simulink model "fin_simu"  (R2022a)
settings: Solver=FixedStepDiscrete  StartTime=0.0  StopTime=time  FixedStep=ts  RelTol=1e-6
values from neighbouring files (symbols this model uses):
  A = [0.7, 0.2; 0, 0.5]    [code_simu.m]    (also in code_simu_continuous.m)
  A0 = [0, 1; -1, -1.4]    [code_simu_continuous.m]
  B = [1; 0.5]    [code_simu.m]    (also in code_simu_continuous.m)
  B0 = [0; 1]    [code_simu_continuous.m]
  C = [0.2, 0.8]    [code_simu.m]    (also in code_simu_continuous.m)
  C0 = [1, 0]    [code_simu_continuous.m]
  D = [0]    [code_simu.m]    (also in code_simu_continuous.m)
  D0 = [0]    [code_simu_continuous.m]
  gamma = 2    [code_simu.m]    (also in code_simu_continuous.m)
  omega = 3.14159265*5    (= 15.70796325)    [code_simu.m]    (also in code_simu_continuous.m)
  ran_max = 20    [code_simu.m]    (also in code_simu_continuous.m)
  ran_min = 5    [code_simu.m]    (also in code_simu_continuous.m)
  rho = 0.101    [code_simu.m]    (also in code_simu_continuous.m)
  sam_time = 40    [code_simu.m]    (also in code_simu_continuous.m)
  seed = 17    [code_simu.m]    (also in code_simu_continuous.m)
  sig = 0.001    [code_simu.m]    (also in code_simu_continuous.m)
  sigma = 10    [code_simu.m]    (also in code_simu_continuous.m)
  ts = 0.005    [code_simu.m]    (also in code_simu_continuous.m)
  wav = 0.7    [code_simu.m]    (also in code_simu_continuous.m)
undefined symbols (not defined in the file or in its folder): A_aspr, AA, b0, b0pfc, b1, b1pfc, b2, b2pfc, b3, b3pfc, B_aspr, BB, C_aspr, CC, D_aspr, DD, w0, w0pfc, w1, w1pfc, w2, w2pfc, w3, w3pfc
libraries: matrix_library x1
settings Model: Creator=lenovo  LastModifiedBy=IDS_PC
settings ModelReferenceCC: EnableRefExpFcnMdlSchedulingChecks=off
settings RTWCC: Description=Generic Real-Time Target  GPUComputeCapability=5.0

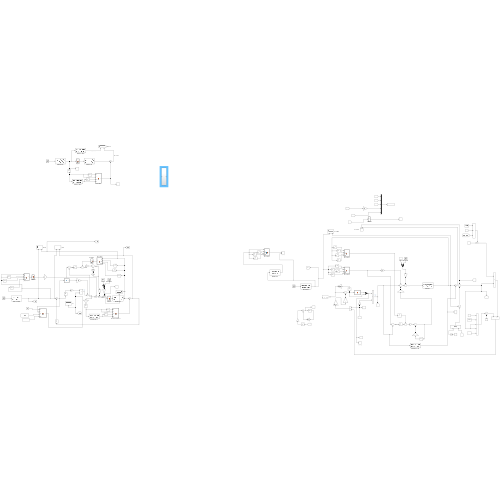
[thumbnail: Simulink's stored preview of the top-level diagram]
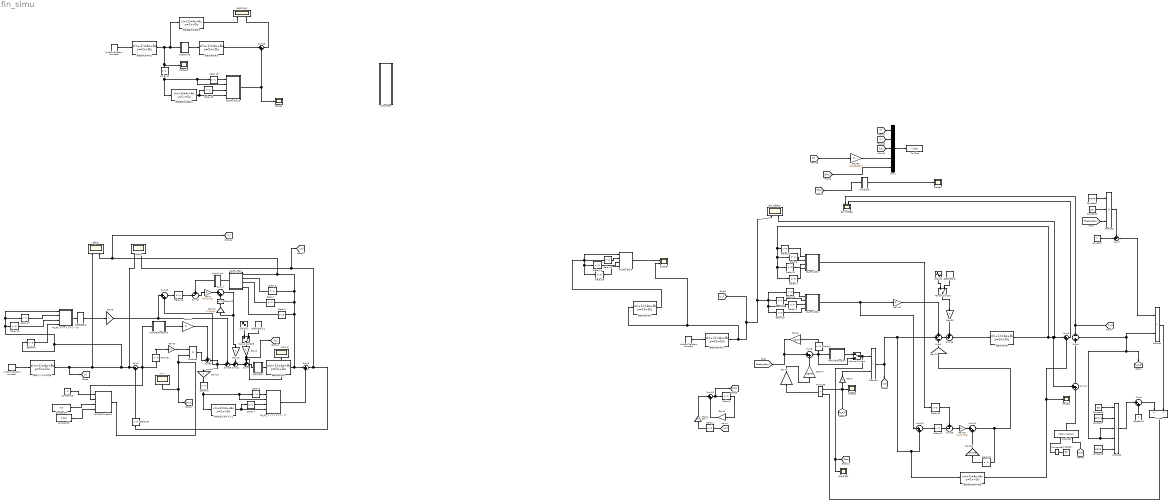
== system fin_simu ==
  " 正弦外乱" : Sin  Amplitude=wav  Frequency=omega  SampleTime=ts
  " 正弦外乱1" : Sin  Amplitude=wav  Frequency=omega  SampleTime=ts
  Constant : Constant  SampleTime=ts
  Constant1 : Constant  Value=sigma  SampleTime=ts
  Constant10 : Constant  Value=0  SampleTime=ts
  Constant14 : Constant  Value=0.5  SampleTime=ts
  Constant15 : Constant  Value=0.001  SampleTime=ts
  Constant2 : Constant  Value=DD  SampleTime=ts
  Constant3 : Constant  Value=sigma  SampleTime=ts
  Constant4 : Constant  SampleTime=ts
  Constant6 : Constant  Value=DD  SampleTime=ts
  Constant7 : Constant  Value=gamma  SampleTime=ts
  Constant8 : Constant  Value=CC  SampleTime=ts
  Delay{1..6,8,12,14,20..23,42..45,47} (18 alike) : Delay  DelayLength=1  InitialCondition=0  SampleTime=ts
  Delay{7,10..11,13,48} (5 alike) : Delay  InitialCondition=0  SampleTime=ts
  Delay{15..16,40,50..51} (5 alike) : Delay  DelayLength=0  InitialCondition=0  SampleTime=ts
  Delay{9,17..19,49} (5 alike) : Delay  DelayLength=3  InitialCondition=0  SampleTime=ts
  Divide : Product  Inputs=/*
  Gain1 : Gain  Gain=BB  Multiplication=Matrix(K*u)
  Gain{5,9..10,12} (4 alike) : Gain
  Gain11 : Gain  Gain=1/(1+sig)
  Gain14 : Gain  Gain=sigma
  Gain{15,21,35,40} (4 alike) : Gain  Gain=0
  Gain2 : Gain  Gain=-1
  Gain3 : Gain  Gain=AA  Multiplication=Matrix(K*u)
  Gain36 : Gain  Gain=1/(1+sig)
  Gain37 : Gain  Gain=rho/(1+sig)
  Gain39 : Gain  Gain=16.66666667
  Gain4 : Gain  Gain=gamma
  Gain6 : Gain  Gain=sigma
  Gain7 : Gain  Gain=rho/(1+sig)
  Gain8 : Gain  Gain=-1
  MATLAB Function : MATLAB Function  TreatAsAtomicUnit=on
  MATLAB Function3 : MATLAB Function  TreatAsAtomicUnit=on
  MATLAB Function4 : MATLAB Function  TreatAsAtomicUnit=on
  Manual Switch1 : ManualSwitch  CurrentSetting=0
  Manual Switch4 : ManualSwitch
  Manual Switch5 : ManualSwitch  CurrentSetting=0
  Mux2 : Mux  Inputs=5
  NNPFC验证 : Scope  NumInputPorts=2
  NN_FF_フィードフォワード7 : MATLAB Function  TreatAsAtomicUnit=on
  NN_FF_フィードフォワード9 : MATLAB Function  TreatAsAtomicUnit=on
  NN_FF_前馈1 : MATLAB Function  TreatAsAtomicUnit=on
  NN_FF_前馈10 : MATLAB Function  TreatAsAtomicUnit=on
  NN_FF_前馈3 : MATLAB Function  TreatAsAtomicUnit=on
  NN_FF_前馈5 : MATLAB Function  TreatAsAtomicUnit=on
  NN_FF_前馈6 : MATLAB Function  TreatAsAtomicUnit=on
  PFC输出 : Scope
  Product{,2,4..5} (4 alike) : Product
  Product1 : Product  Inputs=3
  Product3 : Product  Inputs=5
  Product6 : Product  Multiplication=Matrix(*)
  Scope{1..2,5,10} (4 alike) : Scope
  Subsystem : Subsystem
  Sum1 : Sum  Inputs=|-+
  Sum{4,10,16,28,33} (5 alike) : Sum  Inputs=++|
  Sum11 : Sum  Inputs=-+|
  Sum{2,5,8..9,12..13,15,17,22,24} (10 alike) : Sum  Inputs=|++
  Sum14 : Sum  Inputs=+-|
  Sum23 : Sum  Inputs=+-|
  Sum3 : Sum  Inputs=++-
  Sum6 : Sum  Inputs=-|+
  Sum7 : Sum  Inputs=-+|
  To File2 : ToFile  Filename=linear  MatrixName=linear  SampleTime=ts
  Transpose : matrix_library/Transpose
      settings: SourceProductBaseCode=SL
  Uniform Random Number1 : UniformRandomNumber  Minimum=ran_min  Maximum=ran_max  Seed=seed  SampleTime=sam_time
  Uniform Random Number2 : UniformRandomNumber  Minimum=5  Maximum=20  Seed=seed  SampleTime=sam_time
  Uniform Random Number3 : UniformRandomNumber  Minimum=0  Seed=seed  SampleTime=sam_time
  wailuan : Scope
  ゲイン : Scope
  代号返回器 : MATLAB Function  TreatAsAtomicUnit=on
  伪输出 : Scope  NumInputPorts=2
  拟合效果 : Scope  NumInputPorts=2
  理想拡張正実モデル1 : DiscreteStateSpace  A=A_aspr  B=B_aspr  C=C_aspr  D=D_aspr  SampleTime=ts
  理想概强正实模型2 : DiscreteStateSpace  A=A_aspr  B=B_aspr  C=C_aspr  D=D_aspr  SampleTime=ts
  理想概强正实模型3 : DiscreteStateSpace  A=A_aspr  B=B_aspr  C=C_aspr  D=D_aspr  SampleTime=ts
  真输出1 : Scope  NumInputPorts=2
  离散初始信号机1 : DiscreteStateSpace  A=A0  B=B0  C=C0  D=D0  SampleTime=ts
  离散控制对象 : DiscreteStateSpace  A=A  B=B  C=C  D=D  SampleTime=ts
  离散控制对象2 : DiscreteStateSpace  A=A  B=B  C=C  D=D  SampleTime=ts
  离散控制对象3 : DiscreteStateSpace  A=A  B=B  C=C  D=D  SampleTime=ts
  离散理想前馈补偿器 : DiscreteStateSpace  A=AA  B=BB  C=CC  D=DD  SampleTime=ts
  离散随机信号机1 : DiscreteStateSpace  A=A0  B=B0  C=C0  D=D0  SampleTime=ts
  自适应增益 : Scope
  输入与伪输出 : Scope  NumInputPorts=2
  输入与真输出 : Scope  NumInputPorts=2
  随机阶梯外乱 : UniformRandomNumber  Minimum=-wav  Maximum=wav  Seed=seed+5  SampleTime=16
  随机阶梯外乱1 : UniformRandomNumber  Minimum=-wav  Maximum=wav  Seed=seed+5  SampleTime=16
  離散ランダム信号機 : DiscreteStateSpace  A=A0  B=B0  C=C0  D=D0  SampleTime=ts
  離散制御対象1 : DiscreteStateSpace  A=A  B=B  C=C  D=D  SampleTime=ts
  非線形要素6 : MATLAB Function  TreatAsAtomicUnit=on
  非線形要素7 : MATLAB Function  TreatAsAtomicUnit=on
  非线性元件4 : MATLAB Function  TreatAsAtomicUnit=on
  非线性元件5 : MATLAB Function  TreatAsAtomicUnit=on
  wires:
  Uniform Random Number1/1 -> 离散初始信号机1/1
  Sum6/1 -> Product/2, [e_a_2], Product3/4, Product3/3
  Product1/1 -> Sum7/1
  Constant/1 -> Sum7/2
  Sum7/1 -> Product/1
  Constant1/1 -> Product1/1
  Gain2/1 -> Product4/2
  Sum9/1 -> Manual Switch4/2, Delay2/1, MATLAB Function/1(k)
  Gain6/1 -> Sum9/1, [theta_delay]
  [y_r] -> Sum6/1, 输入与伪输出/1
  Product/1 -> Divide/2
  Sum8/1 -> Divide/1
  Product3/1 -> Sum8/1
  Constant4/1 -> Sum8/2
  Constant7/1 -> Product3/2
  Sum10/1 -> Sum6/2
  [u2] -> Delay1/1
  Delay1/1 -> Gain1/1
  Delay3/1 -> Gain3/1
  Gain3/1 -> Sum12/2
  Sum12/1 -> [xf_k], Delay3/1
  [xf_k] -> Product6/2
  Gain1/1 -> Sum12/1
  Transpose/1 -> Product6/1
  Constant8/1 -> Transpose/1
  Sum5/1 -> Delay50/1, [ya], 伪输出/2
  Uniform Random Number2/1 -> 離散ランダム信号機/1
  離散ランダム信号機/1 -> [r], 伪输出/1, Sum1/1, Delay47/1, NN_FF_フィードフォワード9/1(y), Delay48/1, Delay49/1, 真输出1/1
  [e_a_2] -> Scope5/1, Gain2/1, Product5/1
  [theta_delay] -> Product1/3
  Constant2/1 -> Product1/2
  Constant6/1 -> Product3/1
  Product5/1 -> Gain4/1
  Constant3/1 -> Product3/5
  Gain4/1 -> Gain14/1
  Gain14/1 -> Sum9/2
  Divide/1 -> Product5/2
  Sum16/1 -> 离散控制对象/1  "外乱输入"
  Gain15/1 -> Sum3/1
  Delay2/1 -> Gain6/1
  Product6/1 -> Sum10/2
  Delay8/1 -> NN_FF_前馈3/2(yd)
  Delay10/1 -> NN_FF_前馈3/3(ydd)
  离散控制对象2/1 -> NN_FF_前馈5/1(y), Delay13/1, Delay19/1, Delay14/1
  Delay13/1 -> NN_FF_前馈5/3(ydd)
  Delay14/1 -> NN_FF_前馈5/2(yd)
  NN_FF_前馈5/1(v) -> 拟合效果/1
  Delay15/1 -> NN_FF_前馈3/1(y)
  Delay17/1 -> NN_FF_前馈3/4(yddd)
  Delay16/1 -> NN_FF_前馈6/1(y)
  Delay12/1 -> NN_FF_前馈6/2(yd)
  Delay11/1 -> NN_FF_前馈6/3(ydd)
  Delay18/1 -> NN_FF_前馈6/4(yddd)
  Delay19/1 -> NN_FF_前馈5/4(yddd)
  Manual Switch1/1 -> Gain35/1
  随机阶梯外乱/1 -> Manual Switch1/2
  " 正弦外乱"/1 -> Manual Switch1/1
  离散理想前馈补偿器/1 -> Sum2/2, PFC输出/1
  Sum3/1 -> Sum16/2
  MATLAB Function/1(y) -> Manual Switch4/1
  Product4/1 -> Sum3/2, Sum22/2, 离散理想前馈补偿器/1, [u2]
  离散控制对象/1 -> Delay17/1, Delay10/1, Delay8/1, Delay15/1, Sum2/1, 输入与真输出/2, Sum10/1
  NN_FF_前馈3/1(v) -> Delay40/1
  Gain21/1 -> Sum3/3
  Sum24/1 -> Gain21/1, Delay22/1
  Manual Switch4/1 -> 自适应增益/1, [the], Product4/1
  Sum22/1 -> Delay21/1  "外乱输入"
  Delay21/1 -> Sum23/2
  Sum23/1 -> Gain37/1
  Delay22/1 -> Gain36/1
  离散初始信号机1/1 -> Delay12/1, Delay18/1, Delay11/1, Delay16/1, 输入与真输出/1, [y_r], 拟合效果/2, 离散控制对象2/1
  Delay40/1 -> Sum23/1
  Gain35/1 -> Sum16/1
  NN_FF_前馈6/1(v) -> Sum22/1, Gain15/1
  Gain36/1 -> Sum24/2
  Gain37/1 -> Sum24/1
  非線形要素7/1(y) -> 離散制御対象1/1
  理想拡張正実モデル1/1 -> Delay4/1, NN_FF_フィードフォワード7/4(ya)
  Delay4/1 -> NN_FF_フィードフォワード7/3(ya1)
  Delay5/1 -> NN_FF_フィードフォワード7/1(u1)
  NN_FF_フィードフォワード7/1(v) -> Sum5/2
  Gain8/1 -> Product2/1
  Delay42/1 -> NN_FF_フィードフォワード7/2(u), Delay5/1, 理想拡張正実モデル1/1
  Delay44/1 -> NN_FF_前馈10/2(u), Delay45/1, 理想概强正实模型2/1
  理想概强正实模型2/1 -> NN_FF_前馈10/4(ya), Delay43/1
  Delay43/1 -> NN_FF_前馈10/3(ya1)
  Delay45/1 -> NN_FF_前馈10/1(u1)
  非线性元件5/1(y) -> 离散控制对象3/1
  Uniform Random Number3/1 -> 离散随机信号机1/1
  离散控制对象3/1 -> Sum15/1
  NN_FF_前馈10/1(v) -> Scope2/1, Sum15/2
  理想概强正实模型3/1 -> NNPFC验证/1  "理想扩张输出"
  Sum15/1 -> NNPFC验证/2  "真实扩张输出"
  Mux2/1 -> To File2/1
  [ya] -> Mux2/3
  [r] -> Mux2/1
  [y] -> Mux2/2
  [d] -> Gain39/1
  [the] -> 代号返回器/1(u)
  代号返回器/1(y) -> Scope1/1
  NN_FF_フィードフォワード9/1(v) -> 非線形要素6/1(u)
  Delay47/1 -> NN_FF_フィードフォワード9/2(yd)
  Delay48/1 -> NN_FF_フィードフォワード9/3(ydd)
  Delay49/1 -> NN_FF_フィードフォワード9/4(yddd)
  非線形要素6/1(y) -> Gain9/1
  Gain10/1 -> Delay42/1
  離散制御対象1/1 -> Sum5/1, Delay7/1, [y], 真输出1/2, NN_FF_前馈1/1(y), Delay6/1, Delay9/1
  离散随机信号机1/1 -> Delay44/1, Scope10/1, 理想概强正实模型3/1, 非线性元件5/1(u)
  Delay50/1 -> Sum1/2
  Delay51/1 -> Gain8/1
  Sum2/1 -> 输入与伪输出/2
  Gain39/1 -> Mux2/4
  Constant10/1 -> MATLAB Function4/1(ht)
  Sum1/1 -> MATLAB Function4/2(e), MATLAB Function3/1(e), Delay51/1
  Constant14/1 -> MATLAB Function4/3(sig)
  Constant15/1 -> MATLAB Function4/4(gam)
  MATLAB Function4/1(y) -> ゲイン/1, [thno], Product2/2
  Sum33/1 -> Sum13/2, Sum28/2, Gain10/1
  Product2/1 -> Sum33/2
  MATLAB Function3/1(y) -> Gain40/1
  Gain40/1 -> Sum33/1
  NN_FF_前馈1/1(v) -> 非线性元件4/1(u)
  Manual Switch5/1 -> Gain5/1
  随机阶梯外乱1/1 -> Manual Switch5/2
  " 正弦外乱1"/1 -> Manual Switch5/1
  Sum4/1 -> 非線形要素7/1(u)
  Gain5/1 -> [d], wailuan/1, Sum4/1
  Gain9/1 -> Sum13/1, Sum28/1
  Delay6/1 -> NN_FF_前馈1/2(yd)
  Delay7/1 -> NN_FF_前馈1/3(ydd)
  Delay9/1 -> NN_FF_前馈1/4(yddd)
  Sum11/1 -> Sum4/2  "外乱输入"
  Sum28/1 -> Sum11/2
  Sum13/1 -> Delay20/1  "外乱输入"
  Delay20/1 -> Sum14/2
  非线性元件4/1(y) -> Sum14/1
  Sum14/1 -> Gain7/1  "外乱输入"
  Gain7/1 -> Sum17/1
  Sum17/1 -> Gain12/1, Gain11/1  "外乱输入"
  Gain11/1 -> Delay23/1
  Delay23/1 -> Sum17/2
  Gain12/1 -> Sum11/1
  [thno] -> Mux2/5

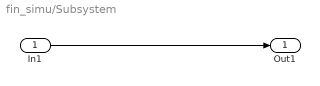
== system fin_simu/Subsystem ==
  In1 : Inport
  Out1 : Outport
  wires:
  In1/1 -> Out1/1

== matlab function fin_simu/NN_FF_フィードフォワード7 ==
  data: u1 input; u input; ya1 input; ya input; v output; w0pfc parameter; w1pfc parameter; w2pfc parameter; w3pfc parameter; b0pfc parameter; b1pfc parameter; b2pfc parameter; b3pfc parameter
function v = fcn(u1, u, ya1, ya, w0pfc, w1pfc, w2pfc, w3pfc, b0pfc, b1pfc, b2pfc, b3pfc)

    x = [ya,ya1,u,u1];
    x = x.';

    s1= (transpose(w0pfc)) * x + b0pfc;
    x1= max(0,s1);     %relu 
    s2= (transpose(w1pfc)) * x1 + b1pfc;
    x2= max(0,s2);     %relu
    s3= (transpose(w2pfc)) * x2 + b2pfc;
    x3= max(0,s3);     %relu
    s4= (transpose(w3pfc)) * x3 + b3pfc;

v=s4;

== matlab function fin_simu/代号返回器 ==
  data: u input; y output
function y = fcn(u)

y = (1+u)/(1-u);
end

== matlab function fin_simu/非线性元件5 ==
  data: u input; y output
function y = fcn(u)

y = 0.06*u^2+0.12*u;
end

== matlab function fin_simu/NN_FF_前馈10 ==
  data: u1 input; u input; ya1 input; ya input; v output; w0pfc parameter; w1pfc parameter; w2pfc parameter; w3pfc parameter; b0pfc parameter; b1pfc parameter; b2pfc parameter; b3pfc parameter
function v = fcn(u1, u, ya1, ya, w0pfc, w1pfc, w2pfc, w3pfc, b0pfc, b1pfc, b2pfc, b3pfc)

    x = [ya,ya1,u,u1];
    x = x.';

    s1= (transpose(w0pfc)) * x + b0pfc;
    x1= max(0,s1);     %relu 
    s2= (transpose(w1pfc)) * x1 + b1pfc;
    x2= max(0,s2);     %relu
    s3= (transpose(w2pfc)) * x2 + b2pfc;
    x3= max(0,s3);     %relu
    s4= (transpose(w3pfc)) * x3 + b3pfc;

v=s4;

== matlab function fin_simu/NN_FF_フィードフォワード9 ==
  data: y input; yd input; ydd input; yddd input; v output; w0 parameter; w1 parameter; w2 parameter; w3 parameter; b0 parameter; b1 parameter; b2 parameter; b3 parameter
function v = fcn(y, yd, ydd, yddd, w0, w1, w2, w3, b0, b1, b2, b3)

    x = [yddd, ydd, yd, y];
    x = x.';

    s1= (transpose(w0)) * x + b0;
    x1= max(0,s1);     %relu 
    s2= (transpose(w1)) * x1 + b1;
    x2= max(0,s2);     %relu
    s3= (transpose(w2)) * x2 + b2;
    x3= max(0,s3);     %relu
    s4= (transpose(w3)) * x3 + b3;

v=s4;

== matlab function fin_simu/非線形要素6 ==
  data: u input; y output
function y = fcn(u)

y = sqrt(u/0.06+1)-1;
end

== matlab function fin_simu/非線形要素7 ==
  data: u input; y output
function y = fcn(u)

y = 0.06*u^2+0.12*u;
end

== matlab function fin_simu/MATLAB Function3 ==
  data: y output; e input
function y = fcn(e)

persistent e_prev;

if isempty(e_prev)
    e_prev = 0;
end

e_next = e_prev + e ;
e_prev = e_next;

y = e_next * 1;

end

== matlab function fin_simu/MATLAB Function4 ==
  data: ht input; y output; e input; sig input; gam input
function y = fcn(ht, e, sig, gam)

persistent k_prev;

if isempty(k_prev)
    k_prev = ht;
end

k_next = k_prev / (1 + sig) + gam / (1 + sig) * e ;
k_prev = k_next;

y = k_next * 1;

end

== matlab function fin_simu/NN_FF_前馈1 ==
  data: y input; yd input; ydd input; yddd input; v output; w0 parameter; w1 parameter; w2 parameter; w3 parameter; b0 parameter; b1 parameter; b2 parameter; b3 parameter
function v = fcn(y, yd, ydd, yddd, w0, w1, w2, w3, b0, b1, b2, b3)

    x = [yddd, ydd, yd, y];
    x = x.';

    s1= (transpose(w0)) * x + b0;
    x1= max(0,s1);     %relu 
    s2= (transpose(w1)) * x1 + b1;
    x2= max(0,s2);     %relu
    s3= (transpose(w2)) * x2 + b2;
    x3= max(0,s3);     %relu
    s4= (transpose(w3)) * x3 + b3;

v=s4;

== matlab function fin_simu/非线性元件4 ==
  data: u input; y output
function y = fcn(u)

y = sqrt(u/0.06+1)-1;
end

== matlab function fin_simu/MATLAB Function ==
  data: y output; k input
function y = fcn(k)

if k>=0 && k<0.999
    y=k;
else
    y=0.998;
end

== matlab function fin_simu/NN_FF_前馈3 ==
  data: y input; yd input; ydd input; yddd input; v output; w0 parameter; w1 parameter; w2 parameter; w3 parameter; b0 parameter; b1 parameter; b2 parameter; b3 parameter
function v = fcn(y, yd, ydd, yddd, w0, w1, w2, w3, b0, b1, b2, b3)

    x = [yddd, ydd, yd, y];
    x = x.';

    s1= (transpose(w0)) * x + b0;
    x1= max(0,s1);     %relu 
    s2= (transpose(w1)) * x1 + b1;
    x2= max(0,s2);     %relu
    s3= (transpose(w2)) * x2 + b2;
    x3= max(0,s3);     %relu
    s4= (transpose(w3)) * x3 + b3;

v=s4;

== matlab function fin_simu/NN_FF_前馈5 ==
  data: y input; yd input; ydd input; yddd input; v output; w0 parameter; w1 parameter; w2 parameter; w3 parameter; b0 parameter; b1 parameter; b2 parameter; b3 parameter
function v = fcn(y, yd, ydd, yddd, w0, w1, w2, w3, b0, b1, b2, b3)

    x = [yddd, ydd, yd, y];
    x = x.';

    s1= (transpose(w0)) * x + b0;
    x1= max(0,s1);     %relu 
    s2= (transpose(w1)) * x1 + b1;
    x2= max(0,s2);     %relu
    s3= (transpose(w2)) * x2 + b2;
    x3= max(0,s3);     %relu
    s4= (transpose(w3)) * x3 + b3;

v=s4;

== matlab function fin_simu/NN_FF_前馈6 ==
  data: y input; yd input; ydd input; yddd input; v output; w0 parameter; w1 parameter; w2 parameter; w3 parameter; b0 parameter; b1 parameter; b2 parameter; b3 parameter
function v = fcn(y, yd, ydd, yddd, w0, w1, w2, w3, b0, b1, b2, b3)

    x = [yddd, ydd, yd, y];
    x = x.';

    s1= (transpose(w0)) * x + b0;
    x1= max(0,s1);     %relu 
    s2= (transpose(w1)) * x1 + b1;
    x2= max(0,s2);     %relu
    s3= (transpose(w2)) * x2 + b2;
    x3= max(0,s3);     %relu
    s4= (transpose(w3)) * x3 + b3;

v=s4;
